simulink model "apll_working"  (R2019b)
settings: Solver=VariableStepAuto  StartTime=0.0  StopTime=1  RelTol=1e-6  AbsTol=1e-6
values from neighbouring files (symbols this model uses):
  G_0 = db2mag(87.3)    [apll_const.m]    (also in attr_for_chaos_generator.m = db2mag(97.7); main.m = db2mag(g); test.m)
  tau_p1 = 1.65*1e-3    (= 0.00165)    [apll_attr.m]    (also in apll_attr_nondim_1.m; apll_attr_nondim_2.m; apll_attr_nondim_3.m; apll_const.m)
  tau_p2 = 1.65*1e-3    (= 0.00165)    [apll_attr.m]    (also in apll_attr_nondim_1.m; apll_attr_nondim_2.m; apll_attr_nondim_3.m; apll_const.m)
  tau_z1 = 165*1e-6    (= 0.000165)    [apll_attr.m]    (also in apll_attr_nondim_1.m; apll_attr_nondim_2.m; apll_attr_nondim_3.m; apll_const.m)
  tau_z2 = 165*1e-6    (= 0.000165)    [apll_attr.m]    (also in apll_attr_nondim_1.m; apll_attr_nondim_2.m; apll_attr_nondim_3.m; apll_const.m)
libraries: simulink x1
settings Model: Creator=Elena  LastModifiedBy=Elena
settings SolverCC: AutoScaleAbsTol=off
settings DebuggingCC: ArithmeticOperatorsInVariantConditions=warning
settings SFSimCC: CustomCodeUndefinedFunction=UseInterfaceOnly
settings CodeAppCC: StateflowObjectComments=on

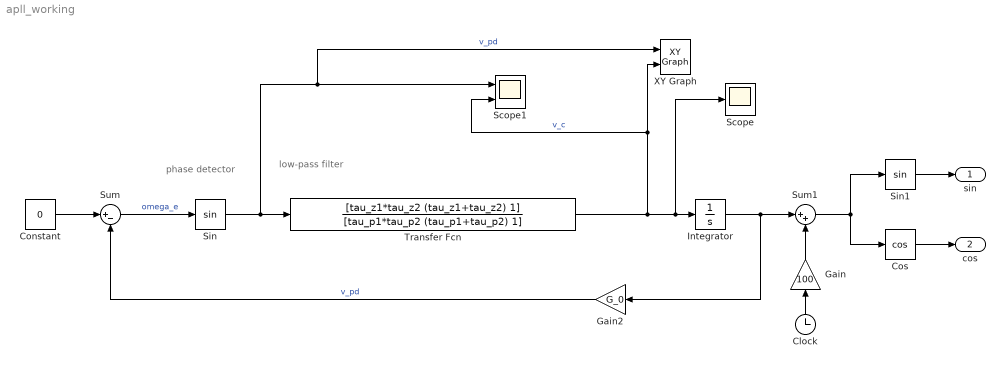
== system apll_working ==
  note: phase detector
  note: low-pass filter
  Clock : Clock
  Constant : Constant  Value=0
  Cos : Trigonometry  Operator=cos
  Gain : Gain  Gain=100
  Gain2 : Gain  Gain=G_0
  Integrator : Integrator  InitialCondition=pi/4
  Scope : Scope
  Scope1 : Scope  NumInputPorts=2
  Sin : Trigonometry
  Sin1 : Trigonometry
  Sum : Sum  Inputs=|+-
  Sum1 : Sum  Inputs=|++
  Transfer Fcn : TransferFcn  Numerator=[tau_z1*tau_z2 (tau_z1+tau_z2) 1]  Denominator=[tau_p1*tau_p2 (tau_p1+tau_p2) 1]
  XY Graph : simulink/Sinks/XY Graph  xmin=-1  xmax=1  ymin=-0.2  ymax=0.2  st=-1
  sin : Outport
  cos : Outport  Port=2
  wires:
  Sum/1 -> Sin/1  "omega_e"
  Constant/1 -> Sum/1
  Cos/1 -> cos/1
  Transfer Fcn/1 -> XY Graph/2, Scope1/2, Scope/1, Integrator/1  "v_c"
  Sin1/1 -> sin/1
  Sin/1 -> Transfer Fcn/1, XY Graph/1, Scope1/1  "v_pd"
  Integrator/1 -> Sum1/1, Gain2/1
  Gain2/1 -> Sum/2  "v_pd"
  Gain/1 -> Sum1/2
  Sum1/1 -> Cos/1, Sin1/1
  Clock/1 -> Gain/1
